simulink model "wurenji"  (R2021a)
settings: Solver=VariableStepAuto  StartTime=0.0  StopTime=10.0  RelTol=1e-3
libraries: pid_lib x4
settings Model: Creator=Administrator  LastModifiedBy=Administrator

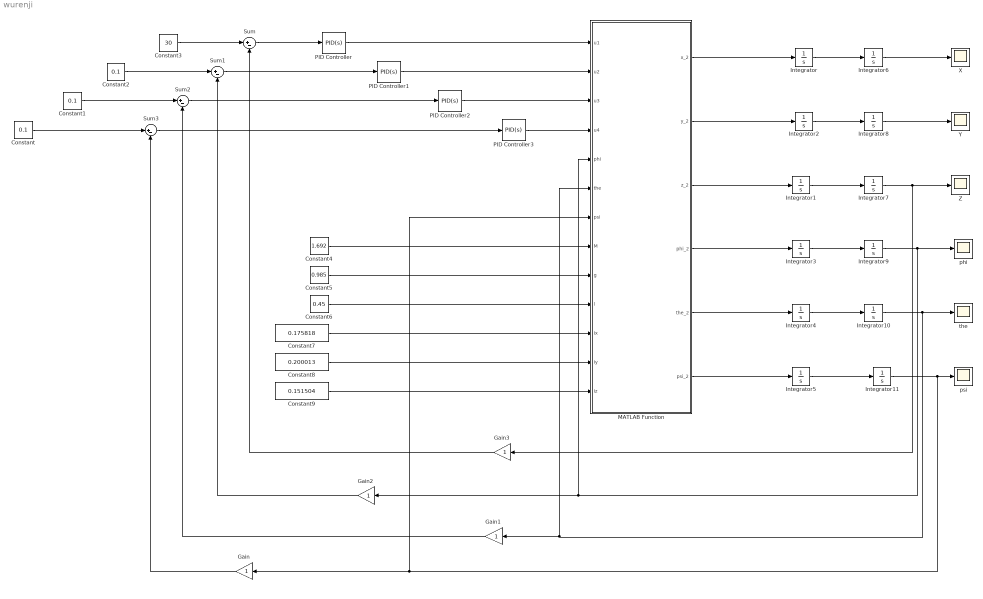
== system wurenji ==
  Constant : Constant  Value=0.1
  Constant1 : Constant  Value=0.1
  Constant2 : Constant  Value=0.1
  Constant3 : Constant  Value=30
  Constant4 : Constant  Value=1.692
  Constant5 : Constant  Value=0.985
  Constant6 : Constant  Value=0.45
  Constant7 : Constant  Value=0.175818
  Constant8 : Constant  Value=0.200013
  Constant9 : Constant  Value=0.151504
  Gain{,1..3} (4 alike) : Gain
  Integrator{,1..11} (12 alike) : Integrator
  MATLAB Function : MATLAB Function  TreatAsAtomicUnit=on
  PID Controller{,1..3} (4 alike) : pid_lib/PID Controller  Controller=PID  Form=Parallel  TimeDomain=Continuous-time  UseExternalTs=off  SampleTime=-1  IntegratorMethod=Forward Euler  FilterMethod=Forward Euler  ControllerParametersSource=internal  P=1  I=1  D=0  UseFilter=on  N=100  TunerSelectOption=Transfer Function Based (PID Tuner App)  InitialConditionSource=internal  InitialConditionForIntegrator=0  InitialConditionForFilter=0  DifferentiatorICPrevScaledInput=0  ExternalReset=none  TrackingMode=off  Kt=1  LimitOutput=off  SatLimitsSource=internal  UpperSaturationLimit=inf  LowerSaturationLimit=-inf  LinearizeAsGain=on  AntiWindupMode=none  Kb=1  POutMin=[]  POutMax=[]  IOutMin=[]  IOutMax=[]  DOutMin=[]  DOutMax=[]  NOutMin=[]  NOutMax=[]  SumOutMin=[]  SumOutMax=[]  SaturationOutMin=[]  SaturationOutMax=[]  PParamMin=[]  PParamMax=[]  IParamMin=[]  IParamMax=[]  DParamMin=[]  DParamMax=[]  NParamMin=[]  NParamMax=[]  KbParamMin=[]  KbParamMax=[]  KtParamMin=[]  KtParamMax=[]  KbOutMin=[]  KbOutMax=[]  KtOutMin=[]  KtOutMax=[]  IntegratorOutMin=[]  IntegratorOutMax=[]  FilterOutMin=[]  FilterOutMax=[]  SumI1OutMin=[]  SumI1OutMax=[]  SumI2OutMin=[]  SumI2OutMax=[]  SumI3OutMin=[]  SumI3OutMax=[]  SumI4OutMin=[]  SumI4OutMax=[]  SumDOutMin=[]  SumDOutMax=[]  DifferentiatorOutMin=[]  DifferentiatorOutMax=[]  FilterDiffOutCoefMin=[]  FilterDiffOutCoefMax=[]  ReciprocalOutMin=[]  ReciprocalOutMax=[]  SumDenOutMin=[]  SumDenOutMax=[]  SumNumOutMin=[]  SumNumOutMax=[]  DivideOutMin=[]  DivideOutMax=[]  UdiffTsProdOutMin=[]  UdiffTsProdOutMax=[]  NTsProdOutMin=[]  NTsProdOutMax=[]  UintegralTsProdOutMin=[]  UintegralTsProdOutMax=[]  UngainTsProdOutMin=[]  UngainTsProdOutMax=[]  IntegratorContinuousStateAttributes=''  IntegratorStateMustResolveToSignalObject=off  IntegratorRTWStateStorageClass=Auto  FilterContinuousStateAttributes=''  FilterStateMustResolveToSignalObject=off  FilterRTWStateStorageClass=Auto  ParallelPVariant=InternalParameters  IdealPVariant=Disabled  IVariant=InternalParameters  DVariant=InternalParameters  IntegratorVariant=Continuous  SatVariant=Disabled  AWVariant=Passthrough  PCopyVariant=Disabled  TRVariant=Disabled  FdbkBlocksVariant=Forward  IdealPFdbkVariant=Disabled  SatFdbkVariant=Disabled  DerivativeFilterVariant=ContFilter  NVariant=InternalParameters  NCopyVariant=Disabled  FilterICVariant=InternalICsFilter  IntegratorICVariant=InternalICs  ExternalResetVariant=Disabled  TRSumVariant=Passthrough  SumFdbkVariant=Disabled  SumVariant=Sum_PID  TsampFilterVariant=InternalTs  TsampNgainVariant=Passthrough  TsampIntegralVariant=Passthrough  ExternalSaturationOutDataTypeStr=Inherit: Same as second input
  Sum{,1..3} (4 alike) : Sum  Inputs=|+-
  X : Scope
  Y : Scope
  Z : Scope
  phi : Scope
  psi : Scope
  the : Scope
  wires:
  Constant3/1 -> Sum/1
  Constant2/1 -> Sum1/1
  Constant1/1 -> Sum2/1
  Constant/1 -> Sum3/1
  Sum/1 -> PID Controller/1
  PID Controller/1 -> MATLAB Function/1(u1)
  Sum1/1 -> PID Controller1/1
  PID Controller1/1 -> MATLAB Function/2(u2)
  Sum2/1 -> PID Controller2/1
  PID Controller2/1 -> MATLAB Function/3(u3)
  Sum3/1 -> PID Controller3/1
  PID Controller3/1 -> MATLAB Function/4(u4)
  Gain/1 -> Sum3/2
  Gain1/1 -> Sum2/2
  Gain2/1 -> Sum1/2
  Gain3/1 -> Sum/2
  MATLAB Function/1(x_2) -> Integrator/1
  Integrator/1 -> Integrator6/1
  MATLAB Function/2(y_2) -> Integrator2/1
  Integrator2/1 -> Integrator8/1
  MATLAB Function/3(z_2) -> Integrator1/1
  Integrator1/1 -> Integrator7/1
  MATLAB Function/4(phi_2) -> Integrator3/1
  Integrator3/1 -> Integrator9/1
  MATLAB Function/5(the_2) -> Integrator4/1
  Integrator4/1 -> Integrator10/1
  MATLAB Function/6(psi_2) -> Integrator5/1
  Integrator5/1 -> Integrator11/1
  Integrator6/1 -> X/1
  Integrator8/1 -> Y/1
  Integrator11/1 -> MATLAB Function/7(psi), Gain/1, psi/1
  Integrator10/1 -> Gain1/1, MATLAB Function/6(the), the/1
  Integrator9/1 -> MATLAB Function/5(phi), Gain2/1, phi/1
  Integrator7/1 -> Gain3/1, Z/1
  Constant4/1 -> MATLAB Function/8(M)
  Constant5/1 -> MATLAB Function/9(g)
  Constant6/1 -> MATLAB Function/10(l)
  Constant7/1 -> MATLAB Function/11(Ix)
  Constant8/1 -> MATLAB Function/12(Iy)
  Constant9/1 -> MATLAB Function/13(Iz)

== matlab function wurenji/MATLAB Function ==
  data: u1 input; x_2 output; u2 input; u3 input; u4 input; phi input; the input; psi input; M input; g input; l input; Ix input; Iy input; Iz input; y_2 output; z_2 output; phi_2 output; the_2 output; psi_2 output
 function [x_2, y_2,z_2,phi_2,the_2,psi_2]=wurenji(u1,u2,u3,u4,phi,the,psi,M,g,l,Ix,Iy,Iz)
x_2=u1*(cos(phi)*sin(the)*cos(psi)+sin(phi)*sin(psi))/M;
y_2=u1*(cos(phi)*sin(the)*cos(psi)-sin(phi)*sin(psi))/M;
z_2=-g+u1*(cos(the)*cos(phi))/M;
phi_2=1*u2/Ix;
the_2=1*u3/Iy;
psi_2=u4*l/Iz;
